simulink model "gm_fourxfour_designfxdpt_givens_vnl"  (R2018b)
settings: Solver=FixedStepDiscrete  StartTime=0.0  StopTime=0.18e-6  RelTol=1e-3
InitFcn:
  | if isempty(which('mylib'))
  |      tmp = fileparts(which(bdroot));
  |      run(fullfile(fileparts(tmp), '5-Utilities', 'addPathsPfcHw.m'));
  | end
  | 
  | data_types_givens
StopFcn:
  | GivensSim_Stop
undefined symbols (not defined in the file or in its folder): f
libraries: simulink x28, mylib x14
(part 1 of 4)
settings Model: Creator=skanaga4  LastModifiedBy=yangli18
settings OptimizationCC: BlockReduction=off  ConditionallyExecuteInputs=off  DefaultParameterBehavior=Inlined
settings DebuggingCC: AlgebraicLoopMsg=error  ArtificialAlgebraicLoopMsg=none  InheritedTsInSrcMsg=none  SingleTaskRateTransMsg=error
settings HardwareCC: ProdBitPerPointer=32  ProdBitPerSizeT=32  ProdBitPerPtrDiffT=32  ProdLargestAtomicFloat=None  ProdIntDivRoundTo=Undefined  ProdEndianess=Unspecified  ProdWordSize=32  ProdHWDeviceType=ASIC/FPGA->ASIC/FPGA  TargetBitPerLong=64  TargetBitPerPointer=64  TargetBitPerSizeT=64  TargetBitPerPtrDiffT=64  TargetLongLongMode=on  TargetIntDivRoundTo=Zero  TargetEndianess=LittleEndian  TargetWordSize=64  TargetHWDeviceType=Custom Processor->MATLAB Host Computer  ProdEqTarget=off

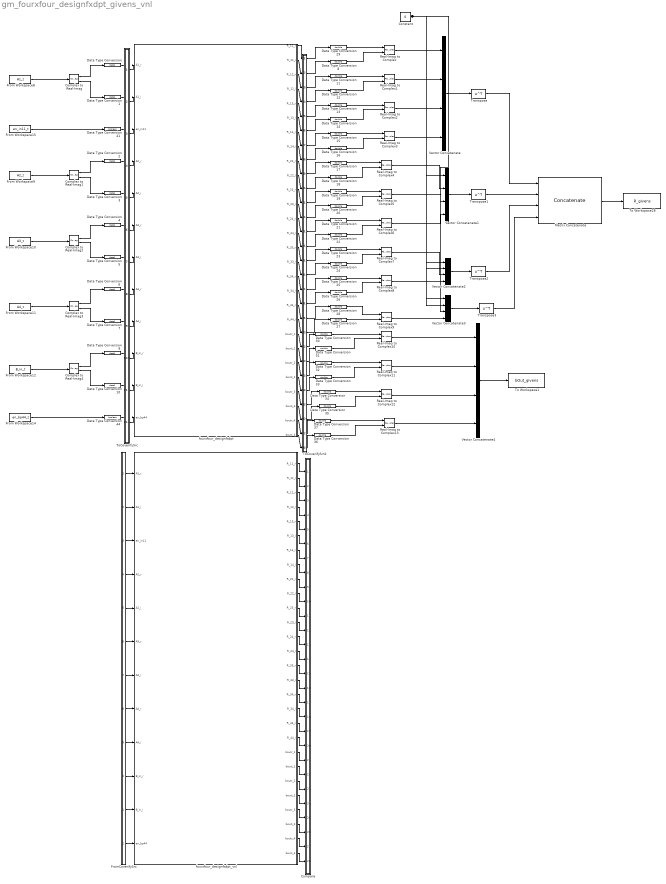
== system gm_fourxfour_designfxdpt_givens_vnl ==
  Compare : Subsystem
      mask Display: disp('')
  Complex to Real-Imag{,1..4} (5 alike) : ComplexToRealImag
  Constant : Constant  Value=0  SampleTime=-1
  Data Type Conversion{,1..7,9..10} (10 alike) : DataTypeConversion  OutDataTypeStr=data1
  Data Type Conversion{8,11..37} (28 alike) : DataTypeConversion  OutDataTypeStr=double
  Data Type Conversion41 : DataTypeConversion  OutDataTypeStr=boolean
  Data Type Conversion44 : DataTypeConversion  OutDataTypeStr=boolean
  From Workspace10 : FromWorkspace  VariableName=A3_t  SampleTime=1/f  Interpolate=off  OutputAfterFinalValue=Holding final value
  From Workspace11 : FromWorkspace  VariableName=A4_t  SampleTime=1/f  Interpolate=off  OutputAfterFinalValue=Holding final value
  From Workspace12 : FromWorkspace  VariableName=B_in_t  SampleTime=1/f  Interpolate=off  OutputAfterFinalValue=Holding final value
  From Workspace14 : FromWorkspace  VariableName=en_bp44_t  SampleTime=1/f  Interpolate=off  OutputAfterFinalValue=Holding final value
  From Workspace15 : FromWorkspace  VariableName=en_in11_t  SampleTime=1/f  Interpolate=off  OutputAfterFinalValue=Holding final value
  From Workspace8 : FromWorkspace  VariableName=A1_t  SampleTime=1/f  Interpolate=off  OutputAfterFinalValue=Holding final value
  From Workspace9 : FromWorkspace  VariableName=A2_t  SampleTime=1/f  Interpolate=off  OutputAfterFinalValue=Holding final value
  FromCoverifySrc : Subsystem
      mask Display: disp('')
  Matrix Concatenate : Concatenate  NumInputs=4  Mode=Multidimensional array
  Real-Imag to Complex{,1..13} (14 alike) : RealImagToComplex
  To Workspace1 : ToWorkspace  VariableName=bOut_givens  SaveFormat=Timeseries  SampleTime=-1
  To Workspace28 : ToWorkspace  VariableName=R_givens  SaveFormat=Timeseries  SampleTime=-1
  ToCoverifySink : Subsystem
      mask Display: disp('')
  ToCoverifySrc : Subsystem
      mask Display: disp('')
  Transpose{,1..3} (4 alike) : Math  Operator=transpose  RndMeth=Zero  SaturateOnIntegerOverflow=on
  Vector Concatenate{,1..4} (5 alike) : Concatenate  NumInputs=4
  fourxfour_designfxdpt : Subsystem
  fourxfour_designfxdpt_vnl : Subsystem
  wires:
  From Workspace8/1 -> Complex to Real-Imag/1
  Complex to Real-Imag/1 -> Data Type Conversion/1
  Complex to Real-Imag/2 -> Data Type Conversion1/1
  From Workspace9/1 -> Complex to Real-Imag1/1
  From Workspace11/1 -> Complex to Real-Imag3/1
  From Workspace10/1 -> Complex to Real-Imag2/1
  Complex to Real-Imag1/1 -> Data Type Conversion2/1
  Complex to Real-Imag1/2 -> Data Type Conversion3/1
  Complex to Real-Imag2/1 -> Data Type Conversion4/1
  Complex to Real-Imag2/2 -> Data Type Conversion5/1
  Complex to Real-Imag3/1 -> Data Type Conversion6/1
  Complex to Real-Imag3/2 -> Data Type Conversion7/1
  From Workspace12/1 -> Complex to Real-Imag4/1
  Complex to Real-Imag4/1 -> Data Type Conversion9/1
  Complex to Real-Imag4/2 -> Data Type Conversion10/1
  From Workspace14/1 -> Data Type Conversion44/1
  From Workspace15/1 -> Data Type Conversion41/1
  Real-Imag to Complex/1 -> Vector Concatenate/1
  Constant/1 -> Vector Concatenate3/3, Vector Concatenate3/2, Vector Concatenate3/1, Vector Concatenate2/2, Vector Concatenate2/1, Vector Concatenate1/1
  Real-Imag to Complex4/1 -> Vector Concatenate1/2
  Real-Imag to Complex9/1 -> Vector Concatenate3/4
  Real-Imag to Complex8/1 -> Vector Concatenate2/4
  Real-Imag to Complex2/1 -> Vector Concatenate/3
  Vector Concatenate/1 -> Transpose/1
  Real-Imag to Complex5/1 -> Vector Concatenate1/3
  Data Type Conversion21/1 -> Real-Imag to Complex6/1
  Data Type Conversion13/1 -> Real-Imag to Complex2/1
  Data Type Conversion12/1 -> Real-Imag to Complex1/2
  Data Type Conversion16/1 -> Real-Imag to Complex3/2
  Data Type Conversion17/1 -> Real-Imag to Complex4/1
  Data Type Conversion18/1 -> Real-Imag to Complex4/2
  Data Type Conversion15/1 -> Real-Imag to Complex3/1
  Data Type Conversion28/1 -> Real-Imag to Complex9/1
  Data Type Conversion29/1 -> Real-Imag to Complex/1
  Matrix Concatenate/1 -> To Workspace28/1
  Vector Concatenate3/1 -> Transpose3/1
  Data Type Conversion23/1 -> Real-Imag to Complex7/1
  Data Type Conversion8/1 -> Real-Imag to Complex/2
  Data Type Conversion24/1 -> Real-Imag to Complex7/2
  Data Type Conversion25/1 -> Real-Imag to Complex8/1
  Transpose/1 -> Matrix Concatenate/1
  Real-Imag to Complex7/1 -> Vector Concatenate2/3
  Transpose3/1 -> Matrix Concatenate/4
  Data Type Conversion19/1 -> Real-Imag to Complex5/1
  Transpose2/1 -> Matrix Concatenate/3
  Data Type Conversion20/1 -> Real-Imag to Complex5/2
  Vector Concatenate1/1 -> Transpose1/1
  Real-Imag to Complex6/1 -> Vector Concatenate1/4
  Transpose1/1 -> Matrix Concatenate/2
  Data Type Conversion22/1 -> Real-Imag to Complex6/2
  Vector Concatenate2/1 -> Transpose2/1
  Data Type Conversion26/1 -> Real-Imag to Complex8/2
  Data Type Conversion11/1 -> Real-Imag to Complex1/1
  Real-Imag to Complex1/1 -> Vector Concatenate/2
  Data Type Conversion14/1 -> Real-Imag to Complex2/2
  Real-Imag to Complex3/1 -> Vector Concatenate/4
  Data Type Conversion27/1 -> Real-Imag to Complex9/2
  Data Type Conversion36/1 -> Real-Imag to Complex13/2
  Data Type Conversion35/1 -> Real-Imag to Complex12/2
  Data Type Conversion31/1 -> Real-Imag to Complex10/2
  Real-Imag to Complex10/1 -> Vector Concatenate4/1
  Real-Imag to Complex11/1 -> Vector Concatenate4/2
  Data Type Conversion34/1 -> Real-Imag to Complex12/1
  Data Type Conversion33/1 -> Real-Imag to Complex11/2
  Data Type Conversion32/1 -> Real-Imag to Complex11/1
  Data Type Conversion37/1 -> Real-Imag to Complex13/1
  Data Type Conversion30/1 -> Real-Imag to Complex10/1
  Real-Imag to Complex12/1 -> Vector Concatenate4/3
  Real-Imag to Complex13/1 -> Vector Concatenate4/4
  Vector Concatenate4/1 -> To Workspace1/1
  ToCoverifySrc/1(out1) -> fourxfour_designfxdpt/1("A1_r ")
  ToCoverifySrc/2(out2) -> fourxfour_designfxdpt/2(A1_i)
  ToCoverifySrc/3(out3) -> fourxfour_designfxdpt/3("en_in11 ")
  ToCoverifySrc/4(out4) -> fourxfour_designfxdpt/4(A2_r)
  ToCoverifySrc/5(out5) -> fourxfour_designfxdpt/5(A2_i)
  ToCoverifySrc/6(out6) -> fourxfour_designfxdpt/6(A3_r)
  ToCoverifySrc/7(out7) -> fourxfour_designfxdpt/7(A3_i)
  ToCoverifySrc/8(out8) -> fourxfour_designfxdpt/8(A4_r)
  ToCoverifySrc/9(out9) -> fourxfour_designfxdpt/9(A4_i)
  ToCoverifySrc/10(out10) -> fourxfour_designfxdpt/10(B_in_r)
  ToCoverifySrc/11(out11) -> fourxfour_designfxdpt/11(B_in_i)
  ToCoverifySrc/12(out12) -> fourxfour_designfxdpt/12(en_bp44)
  fourxfour_designfxdpt/1(R_11_r) -> ToCoverifySink/1(in1)
  fourxfour_designfxdpt/2(R_11_i) -> ToCoverifySink/2(in2)
  fourxfour_designfxdpt/3(R_12_r) -> ToCoverifySink/3(in3)
  fourxfour_designfxdpt/4(R_12_i) -> ToCoverifySink/4(in4)
  fourxfour_designfxdpt/5(R_13_r) -> ToCoverifySink/5(in5)
  fourxfour_designfxdpt/6(R_13_i) -> ToCoverifySink/6(in6)
  fourxfour_designfxdpt/7(R_14_r) -> ToCoverifySink/7(in7)
  fourxfour_designfxdpt/8(R_14_i) -> ToCoverifySink/8(in8)
  fourxfour_designfxdpt/9(R_22_r) -> ToCoverifySink/9(in9)
  fourxfour_designfxdpt/10(R_22_i) -> ToCoverifySink/10(in10)
  fourxfour_designfxdpt/11(R_23_r) -> ToCoverifySink/11(in11)
  fourxfour_designfxdpt/12(R_23_i) -> ToCoverifySink/12(in12)
  fourxfour_designfxdpt/13(R_24_r) -> ToCoverifySink/13(in13)
  fourxfour_designfxdpt/14(R_24_i) -> ToCoverifySink/14(in14)
  fourxfour_designfxdpt/15(R_33_r) -> ToCoverifySink/15(in15)
  fourxfour_designfxdpt/16(R_33_i) -> ToCoverifySink/16(in16)
  fourxfour_designfxdpt/17(R_34_r) -> ToCoverifySink/17(in17)
  fourxfour_designfxdpt/18(R_34_i) -> ToCoverifySink/18(in18)
  fourxfour_designfxdpt/19(R_44_r) -> ToCoverifySink/19(in19)
  fourxfour_designfxdpt/20(R_44_i) -> ToCoverifySink/20(in20)
  fourxfour_designfxdpt/21(boutr_1) -> ToCoverifySink/21(in21)
  fourxfour_designfxdpt/22(bouti_1) -> ToCoverifySink/22(in22)
  fourxfour_designfxdpt/23(boutr_2) -> ToCoverifySink/23(in23)
  fourxfour_designfxdpt/24(bouti_2) -> ToCoverifySink/24(in24)
  fourxfour_designfxdpt/25(boutr_3) -> ToCoverifySink/25(in25)
  fourxfour_designfxdpt/26(bouti_3) -> ToCoverifySink/26(in26)
  fourxfour_designfxdpt/27(boutr_4) -> ToCoverifySink/27(in27)
  fourxfour_designfxdpt/28(bouti_4) -> ToCoverifySink/28(in28)
  Data Type Conversion/1 -> ToCoverifySrc/1(in1)
  Data Type Conversion1/1 -> ToCoverifySrc/2(in2)
  Data Type Conversion41/1 -> ToCoverifySrc/3(in3)
  Data Type Conversion2/1 -> ToCoverifySrc/4(in4)
  Data Type Conversion3/1 -> ToCoverifySrc/5(in5)
  Data Type Conversion4/1 -> ToCoverifySrc/6(in6)
  Data Type Conversion5/1 -> ToCoverifySrc/7(in7)
  Data Type Conversion6/1 -> ToCoverifySrc/8(in8)
  Data Type Conversion7/1 -> ToCoverifySrc/9(in9)
  Data Type Conversion9/1 -> ToCoverifySrc/10(in10)
  Data Type Conversion10/1 -> ToCoverifySrc/11(in11)
  Data Type Conversion44/1 -> ToCoverifySrc/12(in12)
  ToCoverifySink/1(out1) -> Data Type Conversion29/1
  ToCoverifySink/2(out2) -> Data Type Conversion8/1
  ToCoverifySink/3(out3) -> Data Type Conversion11/1
  ToCoverifySink/4(out4) -> Data Type Conversion12/1
  ToCoverifySink/5(out5) -> Data Type Conversion13/1
  ToCoverifySink/6(out6) -> Data Type Conversion14/1
  ToCoverifySink/7(out7) -> Data Type Conversion15/1
  ToCoverifySink/8(out8) -> Data Type Conversion16/1
  ToCoverifySink/9(out9) -> Data Type Conversion17/1
  ToCoverifySink/10(out10) -> Data Type Conversion18/1
  ToCoverifySink/11(out11) -> Data Type Conversion19/1
  ToCoverifySink/12(out12) -> Data Type Conversion20/1
  ToCoverifySink/13(out13) -> Data Type Conversion21/1
  ToCoverifySink/14(out14) -> Data Type Conversion22/1
  ToCoverifySink/15(out15) -> Data Type Conversion23/1
  ToCoverifySink/16(out16) -> Data Type Conversion24/1
  ToCoverifySink/17(out17) -> Data Type Conversion25/1
  ToCoverifySink/18(out18) -> Data Type Conversion26/1
  ToCoverifySink/19(out19) -> Data Type Conversion28/1
  ToCoverifySink/20(out20) -> Data Type Conversion27/1
  ToCoverifySink/21(out21) -> Data Type Conversion30/1
  ToCoverifySink/22(out22) -> Data Type Conversion31/1
  ToCoverifySink/23(out23) -> Data Type Conversion32/1
  ToCoverifySink/24(out24) -> Data Type Conversion33/1
  ToCoverifySink/25(out25) -> Data Type Conversion34/1
  ToCoverifySink/26(out26) -> Data Type Conversion35/1
  ToCoverifySink/27(out27) -> Data Type Conversion37/1
  ToCoverifySink/28(out28) -> Data Type Conversion36/1
  FromCoverifySrc/1(out1) -> fourxfour_designfxdpt_vnl/1("A1_r ")
  FromCoverifySrc/2(out2) -> fourxfour_designfxdpt_vnl/2(A1_i)
  FromCoverifySrc/3(out3) -> fourxfour_designfxdpt_vnl/3("en_in11 ")
  FromCoverifySrc/4(out4) -> fourxfour_designfxdpt_vnl/4(A2_r)
  FromCoverifySrc/5(out5) -> fourxfour_designfxdpt_vnl/5(A2_i)
  FromCoverifySrc/6(out6) -> fourxfour_designfxdpt_vnl/6(A3_r)
  FromCoverifySrc/7(out7) -> fourxfour_designfxdpt_vnl/7(A3_i)
  FromCoverifySrc/8(out8) -> fourxfour_designfxdpt_vnl/8(A4_r)
  FromCoverifySrc/9(out9) -> fourxfour_designfxdpt_vnl/9(A4_i)
  FromCoverifySrc/10(out10) -> fourxfour_designfxdpt_vnl/10(B_in_r)
  FromCoverifySrc/11(out11) -> fourxfour_designfxdpt_vnl/11(B_in_i)
  FromCoverifySrc/12(out12) -> fourxfour_designfxdpt_vnl/12(en_bp44)
  fourxfour_designfxdpt_vnl/1(R_11_r) -> Compare/1(in1)
  fourxfour_designfxdpt_vnl/2(R_11_i) -> Compare/2(in2)
  fourxfour_designfxdpt_vnl/3(R_12_r) -> Compare/3(in3)
  fourxfour_designfxdpt_vnl/4(R_12_i) -> Compare/4(in4)
  fourxfour_designfxdpt_vnl/5(R_13_r) -> Compare/5(in5)
  fourxfour_designfxdpt_vnl/6(R_13_i) -> Compare/6(in6)
  fourxfour_designfxdpt_vnl/7(R_14_r) -> Compare/7(in7)
  fourxfour_designfxdpt_vnl/8(R_14_i) -> Compare/8(in8)
  fourxfour_designfxdpt_vnl/9(R_22_r) -> Compare/9(in9)
  fourxfour_designfxdpt_vnl/10(R_22_i) -> Compare/10(in10)
  fourxfour_designfxdpt_vnl/11(R_23_r) -> Compare/11(in11)
  fourxfour_designfxdpt_vnl/12(R_23_i) -> Compare/12(in12)
  fourxfour_designfxdpt_vnl/13(R_24_r) -> Compare/13(in13)
  fourxfour_designfxdpt_vnl/14(R_24_i) -> Compare/14(in14)
  fourxfour_designfxdpt_vnl/15(R_33_r) -> Compare/15(in15)
  fourxfour_designfxdpt_vnl/16(R_33_i) -> Compare/16(in16)
  fourxfour_designfxdpt_vnl/17(R_34_r) -> Compare/17(in17)
  fourxfour_designfxdpt_vnl/18(R_34_i) -> Compare/18(in18)
  fourxfour_designfxdpt_vnl/19(R_44_r) -> Compare/19(in19)
  fourxfour_designfxdpt_vnl/20(R_44_i) -> Compare/20(in20)
  fourxfour_designfxdpt_vnl/21(boutr_1) -> Compare/21(in21)
  fourxfour_designfxdpt_vnl/22(bouti_1) -> Compare/22(in22)
  fourxfour_designfxdpt_vnl/23(boutr_2) -> Compare/23(in23)
  fourxfour_designfxdpt_vnl/24(bouti_2) -> Compare/24(in24)
  fourxfour_designfxdpt_vnl/25(boutr_3) -> Compare/25(in25)
  fourxfour_designfxdpt_vnl/26(bouti_3) -> Compare/26(in26)
  fourxfour_designfxdpt_vnl/27(boutr_4) -> Compare/27(in27)
  fourxfour_designfxdpt_vnl/28(bouti_4) -> Compare/28(in28)

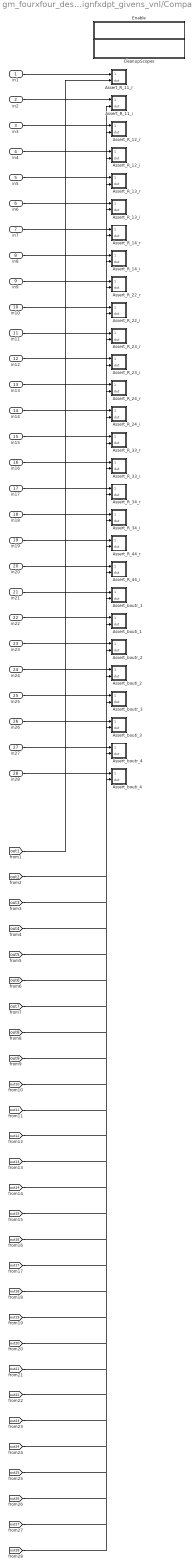
== system gm_fourxfour_designfxdpt_givens_vnl/Compare ==
  in1 : Inport
  in2 : Inport  Port=2
  in3 : Inport  Port=3
  in4 : Inport  Port=4
  in5 : Inport  Port=5
  in6 : Inport  Port=6
  in7 : Inport  Port=7
  in8 : Inport  Port=8
  in9 : Inport  Port=9
  in10 : Inport  Port=10
  in11 : Inport  Port=11
  in12 : Inport  Port=12
  in13 : Inport  Port=13
  in14 : Inport  Port=14
  in15 : Inport  Port=15
  in16 : Inport  Port=16
  in17 : Inport  Port=17
  in18 : Inport  Port=18
  in19 : Inport  Port=19
  in20 : Inport  Port=20
  in21 : Inport  Port=21
  in22 : Inport  Port=22
  in23 : Inport  Port=23
  in24 : Inport  Port=24
  in25 : Inport  Port=25
  in26 : Inport  Port=26
  in27 : Inport  Port=27
  in28 : Inport  Port=28
  Assert_R_11_i : Subsystem
  Assert_R_11_r : Subsystem
  Assert_R_12_i : Subsystem
  Assert_R_12_r : Subsystem
  Assert_R_13_i : Subsystem
  Assert_R_13_r : Subsystem
  Assert_R_14_i : Subsystem
  Assert_R_14_r : Subsystem
  Assert_R_22_i : Subsystem
  Assert_R_22_r : Subsystem
  Assert_R_23_i : Subsystem
  Assert_R_23_r : Subsystem
  Assert_R_24_i : Subsystem
  Assert_R_24_r : Subsystem
  Assert_R_33_i : Subsystem
  Assert_R_33_r : Subsystem
  Assert_R_34_i : Subsystem
  Assert_R_34_r : Subsystem
  Assert_R_44_i : Subsystem
  Assert_R_44_r : Subsystem
  Assert_bouti_1 : Subsystem
  Assert_bouti_2 : Subsystem
  Assert_bouti_3 : Subsystem
  Assert_bouti_4 : Subsystem
  Assert_boutr_1 : Subsystem
  Assert_boutr_2 : Subsystem
  Assert_boutr_3 : Subsystem
  Assert_boutr_4 : Subsystem
  CleanupScopes : Subsystem
      settings: OpenFcn=|
      | blkName = gcb; %self block
      | idx = regexp(blkName, '/CleanupScopes$', 'once');
      | blkParent = blkName(1:idx-1);
      | blks=find_system(blkParent, 'LookUnderMasks', 'all','blocktype', 'Scope');
      | for itr = 1:length(blks)
      | 	 hScopeCfg = get_param(blks{itr},'ScopeConfiguration');
      | 	 hScopeCfg.Visible = ~ hScopeCfg.Visible;
      | end
      | drawnow;
      mask Display: fprintf(message('hdlcoder:cosim:vnl_dblclick').getString());
  Enable : Subsystem
      settings: OpenFcn=|
      | blkName = gcb;
      | idx = regexp(blkName, '/Enable$', 'once');
      | blkParent = blkName(1:idx-1);
      | blks=find_system(blkParent, 'LookUnderMasks', 'all','blocktype', 'Assertion');
      | e = get_param(blks{1}, 'Enabled');
      | if strcmp(e, 'on'), f= 'off';, else, f = 'on';, end
      | for ii=1:length(blks), set_param(blks{ii}, 'Enabled', f);, end
      | set_param(gcb, 'MaskDisplay',['fprintf(message(''hdlcoder:cosim:vnl_dblclick_assertions'',','''',upper(e),'''',').getString())']);
      mask Display: fprintf(message('hdlcoder:cosim:vnl_dblclick_assertions','OFF').getString());
  wires:
  in1/1 -> Assert_R_11_r/1(cosim)
  [out1] -> Assert_R_11_r/2(dut)
  in2/1 -> Assert_R_11_i/1(cosim)
  [out2] -> Assert_R_11_i/2(dut)
  in3/1 -> Assert_R_12_r/1(cosim)
  [out3] -> Assert_R_12_r/2(dut)
  in4/1 -> Assert_R_12_i/1(cosim)
  [out4] -> Assert_R_12_i/2(dut)
  in5/1 -> Assert_R_13_r/1(cosim)
  [out5] -> Assert_R_13_r/2(dut)
  in6/1 -> Assert_R_13_i/1(cosim)
  [out6] -> Assert_R_13_i/2(dut)
  in7/1 -> Assert_R_14_r/1(cosim)
  [out7] -> Assert_R_14_r/2(dut)
  in8/1 -> Assert_R_14_i/1(cosim)
  [out8] -> Assert_R_14_i/2(dut)
  in9/1 -> Assert_R_22_r/1(cosim)
  [out9] -> Assert_R_22_r/2(dut)
  in10/1 -> Assert_R_22_i/1(cosim)
  [out10] -> Assert_R_22_i/2(dut)
  in11/1 -> Assert_R_23_r/1(cosim)
  [out11] -> Assert_R_23_r/2(dut)
  in12/1 -> Assert_R_23_i/1(cosim)
  [out12] -> Assert_R_23_i/2(dut)
  in13/1 -> Assert_R_24_r/1(cosim)
  [out13] -> Assert_R_24_r/2(dut)
  in14/1 -> Assert_R_24_i/1(cosim)
  [out14] -> Assert_R_24_i/2(dut)
  in15/1 -> Assert_R_33_r/1(cosim)
  [out15] -> Assert_R_33_r/2(dut)
  in16/1 -> Assert_R_33_i/1(cosim)
  [out16] -> Assert_R_33_i/2(dut)
  in17/1 -> Assert_R_34_r/1(cosim)
  [out17] -> Assert_R_34_r/2(dut)
  in18/1 -> Assert_R_34_i/1(cosim)
  [out18] -> Assert_R_34_i/2(dut)
  in19/1 -> Assert_R_44_r/1(cosim)
  [out19] -> Assert_R_44_r/2(dut)
  in20/1 -> Assert_R_44_i/1(cosim)
  [out20] -> Assert_R_44_i/2(dut)
  in21/1 -> Assert_boutr_1/1(cosim)
  [out21] -> Assert_boutr_1/2(dut)
  in22/1 -> Assert_bouti_1/1(cosim)
  [out22] -> Assert_bouti_1/2(dut)
  in23/1 -> Assert_boutr_2/1(cosim)
  [out23] -> Assert_boutr_2/2(dut)
  in24/1 -> Assert_bouti_2/1(cosim)
  [out24] -> Assert_bouti_2/2(dut)
  in25/1 -> Assert_boutr_3/1(cosim)
  [out25] -> Assert_boutr_3/2(dut)
  in26/1 -> Assert_bouti_3/1(cosim)
  [out26] -> Assert_bouti_3/2(dut)
  in27/1 -> Assert_boutr_4/1(cosim)
  [out27] -> Assert_boutr_4/2(dut)
  in28/1 -> Assert_bouti_4/1(cosim)
  [out28] -> Assert_bouti_4/2(dut)

== system gm_fourxfour_designfxdpt_givens_vnl/FromCoverifySrc ==
  out1 : Outport
  out2 : Outport  Port=2
  out3 : Outport  Port=3
  out4 : Outport  Port=4
  out5 : Outport  Port=5
  out6 : Outport  Port=6
  out7 : Outport  Port=7
  out8 : Outport  Port=8
  out9 : Outport  Port=9
  out10 : Outport  Port=10
  out11 : Outport  Port=11
  out12 : Outport  Port=12
  wires:
  [in1] -> out1/1
  [in2] -> out2/1
  [in3] -> out3/1
  [in4] -> out4/1
  [in5] -> out5/1
  [in6] -> out6/1
  [in7] -> out7/1
  [in8] -> out8/1
  [in9] -> out9/1
  [in10] -> out10/1
  [in11] -> out11/1
  [in12] -> out12/1

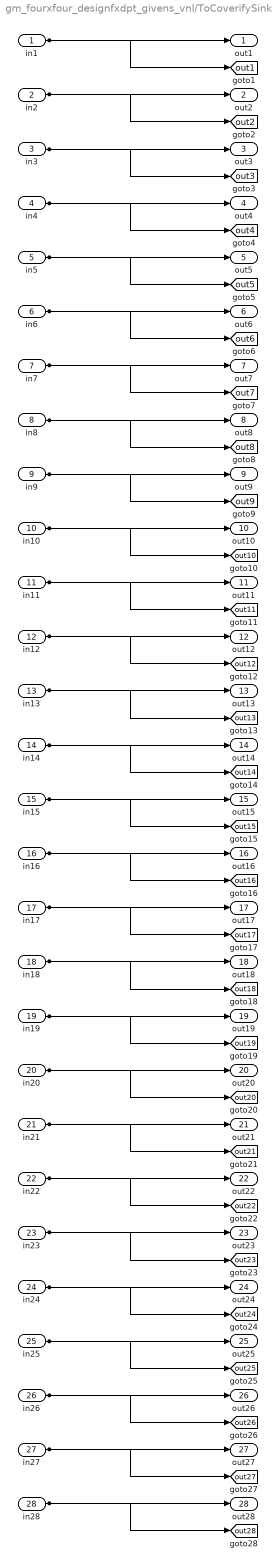
== system gm_fourxfour_designfxdpt_givens_vnl/ToCoverifySink ==
  in1 : Inport
  in2 : Inport  Port=2
  in3 : Inport  Port=3
  in4 : Inport  Port=4
  in5 : Inport  Port=5
  in6 : Inport  Port=6
  in7 : Inport  Port=7
  in8 : Inport  Port=8
  in9 : Inport  Port=9
  in10 : Inport  Port=10
  in11 : Inport  Port=11
  in12 : Inport  Port=12
  in13 : Inport  Port=13
  in14 : Inport  Port=14
  in15 : Inport  Port=15
  in16 : Inport  Port=16
  in17 : Inport  Port=17
  in18 : Inport  Port=18
  in19 : Inport  Port=19
  in20 : Inport  Port=20
  in21 : Inport  Port=21
  in22 : Inport  Port=22
  in23 : Inport  Port=23
  in24 : Inport  Port=24
  in25 : Inport  Port=25
  in26 : Inport  Port=26
  in27 : Inport  Port=27
  in28 : Inport  Port=28
  out1 : Outport
  out2 : Outport  Port=2
  out3 : Outport  Port=3
  out4 : Outport  Port=4
  out5 : Outport  Port=5
  out6 : Outport  Port=6
  out7 : Outport  Port=7
  out8 : Outport  Port=8
  out9 : Outport  Port=9
  out10 : Outport  Port=10
  out11 : Outport  Port=11
  out12 : Outport  Port=12
  out13 : Outport  Port=13
  out14 : Outport  Port=14
  out15 : Outport  Port=15
  out16 : Outport  Port=16
  out17 : Outport  Port=17
  out18 : Outport  Port=18
  out19 : Outport  Port=19
  out20 : Outport  Port=20
  out21 : Outport  Port=21
  out22 : Outport  Port=22
  out23 : Outport  Port=23
  out24 : Outport  Port=24
  out25 : Outport  Port=25
  out26 : Outport  Port=26
  out27 : Outport  Port=27
  out28 : Outport  Port=28
  tag scope: out10=global, out11=global, out12=global, out13=global, out14=global, out15=global, out16=global, out17=global, out18=global, out19=global, out1=global, out20=global, out21=global, out22=global, out23=global, out24=global, out25=global, out26=global, out27=global, out28=global, out2=global, out3=global, out4=global, out5=global, out6=global, out7=global, out8=global, out9=global
  wires:
  in1/1 -> out1/1, [out1]
  in2/1 -> out2/1, [out2]
  in3/1 -> out3/1, [out3]
  in4/1 -> out4/1, [out4]
  in5/1 -> out5/1, [out5]
  in6/1 -> out6/1, [out6]
  in7/1 -> out7/1, [out7]
  in8/1 -> out8/1, [out8]
  in9/1 -> out9/1, [out9]
  in10/1 -> out10/1, [out10]
  in11/1 -> out11/1, [out11]
  in12/1 -> out12/1, [out12]
  in13/1 -> out13/1, [out13]
  in14/1 -> out14/1, [out14]
  in15/1 -> out15/1, [out15]
  in16/1 -> out16/1, [out16]
  in17/1 -> out17/1, [out17]
  in18/1 -> out18/1, [out18]
  in19/1 -> out19/1, [out19]
  in20/1 -> out20/1, [out20]
  in21/1 -> out21/1, [out21]
  in22/1 -> out22/1, [out22]
  in23/1 -> out23/1, [out23]
  in24/1 -> out24/1, [out24]
  in25/1 -> out25/1, [out25]
  in26/1 -> out26/1, [out26]
  in27/1 -> out27/1, [out27]
  in28/1 -> out28/1, [out28]

== system gm_fourxfour_designfxdpt_givens_vnl/ToCoverifySrc ==
  in1 : Inport
  in2 : Inport  Port=2
  in3 : Inport  Port=3
  in4 : Inport  Port=4
  in5 : Inport  Port=5
  in6 : Inport  Port=6
  in7 : Inport  Port=7
  in8 : Inport  Port=8
  in9 : Inport  Port=9
  in10 : Inport  Port=10
  in11 : Inport  Port=11
  in12 : Inport  Port=12
  out1 : Outport
  out2 : Outport  Port=2
  out3 : Outport  Port=3
  out4 : Outport  Port=4
  out5 : Outport  Port=5
  out6 : Outport  Port=6
  out7 : Outport  Port=7
  out8 : Outport  Port=8
  out9 : Outport  Port=9
  out10 : Outport  Port=10
  out11 : Outport  Port=11
  out12 : Outport  Port=12
  tag scope: in10=global, in11=global, in12=global, in1=global, in2=global, in3=global, in4=global, in5=global, in6=global, in7=global, in8=global, in9=global
  wires:
  in1/1 -> out1/1, [in1]
  in2/1 -> out2/1, [in2]
  in3/1 -> out3/1, [in3]
  in4/1 -> out4/1, [in4]
  in5/1 -> out5/1, [in5]
  in6/1 -> out6/1, [in6]
  in7/1 -> out7/1, [in7]
  in8/1 -> out8/1, [in8]
  in9/1 -> out9/1, [in9]
  in10/1 -> out10/1, [in10]
  in11/1 -> out11/1, [in11]
  in12/1 -> out12/1, [in12]

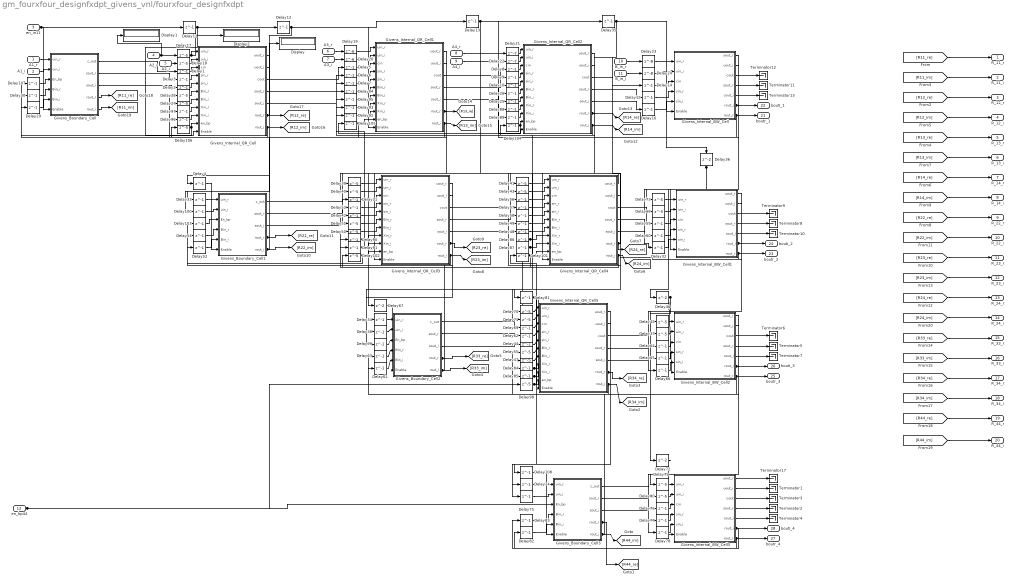
== system gm_fourxfour_designfxdpt_givens_vnl/fourxfour_designfxdpt ==
  "A1_r " : Inport  OutDataTypeStr=fixdt(1, 24, 14)  PortDimensions=1  SampleTime=1e-08
  A1_i : Inport  Port=2  OutDataTypeStr=fixdt(1, 24, 14)  PortDimensions=1  SampleTime=1e-08
  "en_in11 " : Inport  Port=3  OutDataTypeStr=boolean  PortDimensions=1  SampleTime=1e-08
  A2_r : Inport  Port=4  OutDataTypeStr=fixdt(1, 24, 14)  PortDimensions=1  SampleTime=1e-08
  A2_i : Inport  Port=5  OutDataTypeStr=fixdt(1, 24, 14)  PortDimensions=1  SampleTime=1e-08
  A3_r : Inport  Port=6  OutDataTypeStr=fixdt(1, 24, 14)  PortDimensions=1  SampleTime=1e-08
  A3_i : Inport  Port=7  OutDataTypeStr=fixdt(1, 24, 14)  PortDimensions=1  SampleTime=1e-08
  A4_r : Inport  Port=8  OutDataTypeStr=fixdt(1, 24, 14)  PortDimensions=1  SampleTime=1e-08
  A4_i : Inport  Port=9  OutDataTypeStr=fixdt(1, 24, 14)  PortDimensions=1  SampleTime=1e-08
  B_in_r : Inport  Port=10  OutDataTypeStr=fixdt(1, 24, 14)  PortDimensions=1  SampleTime=1e-08
  B_in_i : Inport  Port=11  OutDataTypeStr=fixdt(1, 24, 14)  PortDimensions=1  SampleTime=1e-08
  en_bp44 : Inport  Port=12  OutDataTypeStr=boolean  PortDimensions=1  SampleTime=1e-08
  Delay{1..16,25..26,29..35,38,42,44,48..49,52..54,56..66,69,74..78,81..97,99..101,103..105,107..108} (75 alike) : Delay  DelayLength=1  InitialCondition=0
  Delay{17..18,27..28,37,39..41,43,45,47,50..51,55,68,70..71,73,79..80,98,102,106} (23 alike) : Delay  DelayLength=5  InitialCondition=0
  Delay19 : Delay  DelayLength=6  InitialCondition=0
  Delay20 : Delay  DelayLength=6  InitialCondition=0
  Delay21 : Delay  DelayLength=7  InitialCondition=0
  Delay22 : Delay  DelayLength=7  InitialCondition=0
  Delay23 : Delay  DelayLength=8  InitialCondition=0
  Delay24 : Delay  DelayLength=8  InitialCondition=0
  Delay{36,46,67,72} (4 alike) : Delay  InitialCondition=0
  Display : Display
  Display1 : Display
  Display2 : Display
  Givens_Boundary_Cell : Subsystem
  Givens_Boundary_Cell1 : Subsystem
  Givens_Boundary_Cell2 : Subsystem
  Givens_Boundary_Cell3 : Subsystem
  Givens_Internal_BW_Cell : Subsystem
  Givens_Internal_BW_Cell1 : Subsystem
  Givens_Internal_BW_Cell2 : Subsystem
  Givens_Internal_BW_Cell3 : Subsystem
  Givens_Internal_QR_Cell : Subsystem
  Givens_Internal_QR_Cell1 : Subsystem
  Givens_Internal_QR_Cell2 : Subsystem
  Givens_Internal_QR_Cell3 : Subsystem
  Givens_Internal_QR_Cell4 : Subsystem
  Givens_Internal_QR_Cell5 : Subsystem
  Terminator{1..13,17} (14 alike) : Terminator
  R_11_r : Outport
  R_11_i : Outport  Port=2
  R_12_r : Outport  Port=3
  R_12_i : Outport  Port=4
  R_13_r : Outport  Port=5
  R_13_i : Outport  Port=6
  R_14_r : Outport  Port=7
  R_14_i : Outport  Port=8
  R_22_r : Outport  Port=9
  R_22_i : Outport  Port=10
  R_23_r : Outport  Port=11
  R_23_i : Outport  Port=12
  R_24_r : Outport  Port=13
  R_24_i : Outport  Port=14
  R_33_r : Outport  Port=15
  R_33_i : Outport  Port=16
  R_34_r : Outport  Port=17
  R_34_i : Outport  Port=18
  R_44_r : Outport  Port=19
  R_44_i : Outport  Port=20
  boutr_1 : Outport  Port=21
  bouti_1 : Outport  Port=22
  boutr_2 : Outport  Port=23
  bouti_2 : Outport  Port=24
  boutr_3 : Outport  Port=25
  bouti_3 : Outport  Port=26
  boutr_4 : Outport  Port=27
  bouti_4 : Outport  Port=28
  wires:
  Givens_Boundary_Cell/3(sout_i) -> Delay2/1
  Givens_Boundary_Cell/2(sout_r) -> Delay3/1
  Givens_Boundary_Cell/1(c_out) -> Delay1/1
  Givens_Internal_QR_Cell/5(sout_i) -> Delay7/1
  Givens_Internal_QR_Cell/4(sout_r) -> Delay6/1
  Givens_Internal_QR_Cell/3(cout) -> Delay5/1
  Givens_Internal_QR_Cell/2(uout_i) -> Delay100/1
  Givens_Internal_QR_Cell/1(uout_r) -> Delay33/1
  Delay1/1 -> Givens_Internal_QR_Cell/3(cin)
  Delay3/1 -> Givens_Internal_QR_Cell/4(sin_r)
  Delay2/1 -> Givens_Internal_QR_Cell/5(sin_i)
  Givens_Internal_QR_Cell1/5(sout_i) -> Delay10/1
  Givens_Internal_QR_Cell1/4(sout_r) -> Delay9/1
  Givens_Internal_QR_Cell1/3(cout) -> Delay8/1
  Givens_Internal_QR_Cell1/2(uout_i) -> Delay40/1
  Givens_Internal_QR_Cell1/1(uout_r) -> Delay39/1
  Delay5/1 -> Givens_Internal_QR_Cell1/3(cin)
  Delay6/1 -> Givens_Internal_QR_Cell1/4(sin_r)
  Delay7/1 -> Givens_Internal_QR_Cell1/5(sin_i)
  Givens_Internal_QR_Cell2/5(sout_i) -> Delay16/1
  Givens_Internal_QR_Cell2/4(sout_r) -> Delay15/1
  Givens_Internal_QR_Cell2/3(cout) -> Delay14/1
  Givens_Internal_QR_Cell2/2(uout_i) -> Delay43/1
  Givens_Internal_QR_Cell2/1(uout_r) -> Delay41/1
  Delay8/1 -> Givens_Internal_QR_Cell2/3(cin)
  Delay9/1 -> Givens_Internal_QR_Cell2/4(sin_r)
  Delay10/1 -> Givens_Internal_QR_Cell2/5(sin_i)
  Givens_Internal_BW_Cell/2(uout_i) -> Delay68/1
  Givens_Internal_BW_Cell/1(uout_r) -> Delay73/1
  Delay14/1 -> Givens_Internal_BW_Cell/3(cin)
  Delay15/1 -> Givens_Internal_BW_Cell/4(sin_r)
  Delay16/1 -> Givens_Internal_BW_Cell/5(sin_i)
  Delay26/1 -> Givens_Internal_QR_Cell2/6(Bin_r)
  Delay25/1 -> Givens_Internal_QR_Cell2/7(Bin_i)
  Givens_Boundary_Cell3/3(sout_i) -> Delay78/1
  Givens_Boundary_Cell3/2(sout_r) -> Delay77/1
  Givens_Boundary_Cell3/1(c_out) -> Delay76/1
  Givens_Internal_QR_Cell5/5(sout_i) -> Delay66/1
  Givens_Internal_QR_Cell5/4(sout_r) -> Delay65/1
  Givens_Internal_QR_Cell5/3(cout) -> Delay64/1
  Givens_Internal_QR_Cell5/2(uout_i) -> Delay75/1
  Givens_Internal_QR_Cell5/1(uout_r) -> Delay74/1
  Givens_Internal_QR_Cell4/5(sout_i) -> Delay32/1
  Givens_Internal_QR_Cell4/4(sout_r) -> Delay60/1
  Givens_Internal_QR_Cell4/3(cout) -> Delay59/1
  Givens_Internal_QR_Cell4/2(uout_i) -> Delay71/1
  Givens_Internal_QR_Cell4/1(uout_r) -> Delay70/1
  Delay41/1 -> Givens_Internal_QR_Cell4/1(uin_r)
  Delay43/1 -> Givens_Internal_QR_Cell4/2(uin_i)
  Givens_Internal_QR_Cell3/5(sout_i) -> Delay58/1
  Givens_Internal_QR_Cell3/4(sout_r) -> Delay57/1
  Givens_Internal_QR_Cell3/3(cout) -> Delay56/1
  Givens_Internal_QR_Cell3/2(uout_i) -> Delay38/1
  Givens_Internal_QR_Cell3/1(uout_r) -> Delay34/1
  Delay39/1 -> Givens_Internal_QR_Cell3/1(uin_r)
  Delay40/1 -> Givens_Internal_QR_Cell3/2(uin_i)
  Givens_Boundary_Cell1/3(sout_i) -> Delay42/1
  Givens_Boundary_Cell1/2(sout_r) -> Delay53/1
  Givens_Boundary_Cell1/1(c_out) -> Delay31/1
  Delay33/1 -> Givens_Boundary_Cell1/1(uin_r)
  Delay100/1 -> Givens_Boundary_Cell1/2(uin_i)
  Delay54/1 -> Givens_Boundary_Cell1/4(Bin_r)
  Delay52/1 -> Givens_Boundary_Cell1/5(Bin_i)
  Delay31/1 -> Givens_Internal_QR_Cell3/3(cin)
  Delay53/1 -> Givens_Internal_QR_Cell3/4(sin_r)
  Delay42/1 -> Givens_Internal_QR_Cell3/5(sin_i)
  Delay51/1 -> Givens_Internal_QR_Cell3/6(Bin_r)
  Delay50/1 -> Givens_Internal_QR_Cell3/7(Bin_i)
  Givens_Boundary_Cell2/3(sout_i) -> Delay44/1
  Givens_Boundary_Cell2/2(sout_r) -> Delay62/1
  Givens_Boundary_Cell2/1(c_out) -> Delay69/1
  Delay34/1 -> Givens_Boundary_Cell2/1(uin_r)
  Delay38/1 -> Givens_Boundary_Cell2/2(uin_i)
  Delay63/1 -> Givens_Boundary_Cell2/4(Bin_r)
  Delay61/1 -> Givens_Boundary_Cell2/5(Bin_i)
  Delay90/1 -> Givens_Internal_QR_Cell3/8(Xin_r), Delay93/1
  Delay91/1 -> Givens_Internal_QR_Cell3/9(Xin_i), Delay92/1
  Delay56/1 -> Givens_Internal_QR_Cell4/3(cin)
  Delay57/1 -> Givens_Internal_QR_Cell4/4(sin_r)
  Delay58/1 -> Givens_Internal_QR_Cell4/5(sin_i)
  Givens_Internal_BW_Cell1/2(uout_i) -> Delay37/1
  Givens_Internal_BW_Cell1/1(uout_r) -> Delay45/1
  Delay73/1 -> Givens_Internal_BW_Cell1/1(uin_r)
  Delay68/1 -> Givens_Internal_BW_Cell1/2(uin_i)
  Delay59/1 -> Givens_Internal_BW_Cell1/3(cin)
  Delay60/1 -> Givens_Internal_BW_Cell1/4(sin_r)
  Delay32/1 -> Givens_Internal_BW_Cell1/5(sin_i)
  Delay49/1 -> Givens_Internal_QR_Cell4/6(Bin_r)
  Delay48/1 -> Givens_Internal_QR_Cell4/7(Bin_i)
  Delay86/1 -> Givens_Internal_QR_Cell4/8(Xin_r), Delay88/1
  Delay84/1 -> Givens_Internal_QR_Cell5/8(Xin_r), Delay86/1
  Delay85/1 -> Givens_Internal_QR_Cell5/9(Xin_i), Delay87/1
  Delay87/1 -> Givens_Internal_QR_Cell4/9(Xin_i), Delay89/1
  Delay70/1 -> Givens_Internal_QR_Cell5/1(uin_r)
  Delay71/1 -> Givens_Internal_QR_Cell5/2(uin_i)
  Delay69/1 -> Givens_Internal_QR_Cell5/3(cin)
  Delay62/1 -> Givens_Internal_QR_Cell5/4(sin_r)
  Delay44/1 -> Givens_Internal_QR_Cell5/5(sin_i)
  Givens_Internal_BW_Cell2/2(uout_i) -> Delay80/1
  Givens_Internal_BW_Cell2/1(uout_r) -> Delay79/1
  Delay45/1 -> Givens_Internal_BW_Cell2/1(uin_r)
  Delay37/1 -> Givens_Internal_BW_Cell2/2(uin_i)
  Delay64/1 -> Givens_Internal_BW_Cell2/3(cin)
  Delay65/1 -> Givens_Internal_BW_Cell2/4(sin_r)
  Delay66/1 -> Givens_Internal_BW_Cell2/5(sin_i)
  Delay55/1 -> Givens_Internal_QR_Cell5/6(Bin_r)
  Delay47/1 -> Givens_Internal_QR_Cell5/7(Bin_i)
  Delay74/1 -> Givens_Boundary_Cell3/1(uin_r)
  Delay75/1 -> Givens_Boundary_Cell3/2(uin_i)
  Delay79/1 -> Givens_Internal_BW_Cell3/1(uin_r)
  Delay80/1 -> Givens_Internal_BW_Cell3/2(uin_i)
  Delay76/1 -> Givens_Internal_BW_Cell3/3(cin)
  Delay77/1 -> Givens_Internal_BW_Cell3/4(sin_r)
  Delay78/1 -> Givens_Internal_BW_Cell3/5(sin_i)
  Delay83/1 -> Givens_Boundary_Cell3/4(Bin_r)
  Delay82/1 -> Givens_Boundary_Cell3/5(Bin_i)
  Delay88/1 -> Givens_Internal_QR_Cell2/8(Xin_r)
  Delay89/1 -> Givens_Internal_QR_Cell2/9(Xin_i)
  Delay94/1 -> Givens_Internal_QR_Cell1/6(Bin_r)
  Delay95/1 -> Givens_Internal_QR_Cell1/7(Bin_i)
  Delay93/1 -> Givens_Internal_QR_Cell1/8(Xin_r)
  Delay92/1 -> Givens_Internal_QR_Cell1/9(Xin_i)
  Delay28/1 -> Givens_Internal_QR_Cell/6(Bin_r)
  Delay27/1 -> Givens_Internal_QR_Cell/7(Bin_i)
  Delay97/1 -> Givens_Internal_QR_Cell/8(Xin_r)
  Delay96/1 -> Givens_Internal_QR_Cell/9(Xin_i)
  Delay30/1 -> Givens_Boundary_Cell/4(Bin_r)
  Delay29/1 -> Givens_Boundary_Cell/5(Bin_i)
  Givens_Internal_QR_Cell5/7(rout_i) -> Delay61/1, [R34_im]
  Givens_Internal_QR_Cell5/6(rout_r) -> Delay63/1, [R34_re]
  Givens_Internal_QR_Cell4/7(rout_i) -> Delay50/1, [R24_im]
  Givens_Internal_QR_Cell4/6(rout_r) -> Delay51/1, [R24_re]
  Givens_Internal_QR_Cell3/7(rout_i) -> Delay52/1, [R23_im]
  Givens_Internal_QR_Cell3/6(rout_r) -> Delay54/1, [R23_re]
  Givens_Internal_QR_Cell2/7(rout_i) -> Delay95/1, [R14_im]
  Givens_Internal_QR_Cell2/6(rout_r) -> Delay94/1, [R14_re]
  Givens_Internal_QR_Cell1/7(rout_i) -> Delay27/1, [R13_im]
  Givens_Internal_QR_Cell1/6(rout_r) -> Delay28/1, [R13_re]
  Givens_Internal_QR_Cell/7(rout_i) -> Delay29/1, [R12_im]
  Givens_Internal_QR_Cell/6(rout_r) -> Delay30/1, Display/1, [R12_re]
  Givens_Internal_BW_Cell3/7(rout_r) -> Delay83/1, boutr_4/1
  Givens_Internal_BW_Cell3/6(rout_i) -> Delay82/1, bouti_4/1
  Givens_Internal_BW_Cell3/5(sout_i) -> Terminator4/1
  Givens_Internal_BW_Cell3/4(sout_r) -> Terminator2/1
  Givens_Internal_BW_Cell3/3(cout) -> Terminator3/1
  Givens_Internal_BW_Cell3/2(uout_i) -> Terminator1/1
  Givens_Internal_BW_Cell3/1(uout_r) -> Terminator17/1
  Givens_Internal_BW_Cell2/7(rout_r) -> Delay55/1, boutr_3/1
  Givens_Internal_BW_Cell2/6(rout_i) -> Delay47/1, bouti_3/1
  Givens_Internal_BW_Cell2/5(sout_i) -> Terminator7/1
  Givens_Internal_BW_Cell2/4(sout_r) -> Terminator5/1
  Givens_Internal_BW_Cell2/3(cout) -> Terminator6/1
  Givens_Internal_BW_Cell1/7(rout_r) -> Delay49/1, boutr_2/1
  Givens_Internal_BW_Cell1/6(rout_i) -> Delay48/1, bouti_2/1
  Givens_Internal_BW_Cell1/5(sout_i) -> Terminator10/1
  Givens_Internal_BW_Cell1/4(sout_r) -> Terminator8/1
  Givens_Internal_BW_Cell1/3(cout) -> Terminator9/1
  Givens_Internal_BW_Cell/7(rout_r) -> Delay26/1, boutr_1/1
  Givens_Internal_BW_Cell/6(rout_i) -> Delay25/1, bouti_1/1
  Givens_Internal_BW_Cell/5(sout_i) -> Terminator13/1
  Givens_Internal_BW_Cell/4(sout_r) -> Terminator11/1
  Givens_Internal_BW_Cell/3(cout) -> Terminator12/1
  Givens_Boundary_Cell3/5(rout_i) -> Delay85/1, [R44_im]
  Givens_Boundary_Cell3/4(rout_r) -> Delay84/1, [R44_re]
  Givens_Boundary_Cell2/5(rout_i) -> Delay91/1, [R33_im]
  Givens_Boundary_Cell2/4(rout_r) -> Delay90/1, [R33_re]
  Givens_Boundary_Cell1/5(rout_i) -> Delay96/1, [R22_im]
  Givens_Boundary_Cell1/4(rout_r) -> Delay97/1, [R22_re]
  Givens_Boundary_Cell/5(rout_i) -> [R11_im]
  Givens_Boundary_Cell/4(rout_r) -> [R11_re]
  [R14_im] -> R_14_i/1
  [R22_re] -> R_22_r/1
  [R13_im] -> R_13_i/1
  [R14_re] -> R_14_r/1
  [R12_im] -> R_12_i/1
  [R13_re] -> R_13_r/1
  [R11_im] -> R_11_i/1
  [R24_im] -> R_24_i/1
  [R12_re] -> R_12_r/1
  [R44_im] -> R_44_i/1
  [R44_re] -> R_44_r/1
  [R34_im] -> R_34_i/1
  [R34_re] -> R_34_r/1
  [R33_im] -> R_33_i/1
  [R33_re] -> R_33_r/1
  [R23_im] -> R_23_i/1
  [R24_re] -> R_24_r/1
  [R22_im] -> R_22_i/1
  [R23_re] -> R_23_r/1
  [R11_re] -> R_11_r/1
  Delay99/1 -> Givens_Boundary_Cell2/3(En_bp)
  Delay98/1 -> Givens_Internal_QR_Cell5/10(en_bp), Delay101/1, Delay99/1
  Delay81/1 -> Givens_Internal_QR_Cell5/11(Enable), Delay108/1
  Delay72/1 -> Givens_Internal_BW_Cell3/6(Enable)
  Delay67/1 -> Givens_Boundary_Cell2/6(Enable)
  Delay46/1 -> Givens_Internal_BW_Cell2/6(Enable), Delay72/1
  Delay4/1 -> Givens_Boundary_Cell1/6(Enable)
  Delay36/1 -> Givens_Internal_BW_Cell1/6(Enable), Delay46/1
  Delay35/1 -> Givens_Internal_BW_Cell/6(Enable), Givens_Internal_QR_Cell4/11(Enable), Delay36/1, Delay67/1, Delay81/1
  Delay24/1 -> Givens_Internal_BW_Cell/2(uin_i)
  Delay23/1 -> Givens_Internal_BW_Cell/1(uin_r)
  Delay22/1 -> Givens_Internal_QR_Cell2/2(uin_i)
  Delay21/1 -> Givens_Internal_QR_Cell2/1(uin_r)
  Delay20/1 -> Givens_Internal_QR_Cell1/2(uin_i)
  Delay19/1 -> Givens_Internal_QR_Cell1/1(uin_r)
  Delay18/1 -> Givens_Internal_QR_Cell/2(uin_i)
  Delay17/1 -> Givens_Internal_QR_Cell/1(uin_r), Display2/1
  Delay13/1 -> Givens_Internal_QR_Cell3/11(Enable), Givens_Internal_QR_Cell2/11(Enable), Delay35/1
  Delay12/1 -> Givens_Internal_QR_Cell1/11(Enable), Delay13/1, Delay4/1
  Delay11/1 -> Givens_Internal_QR_Cell/11(Enable), Delay12/1
  Delay108/1 -> Givens_Boundary_Cell3/6(Enable)
  Delay107/1 -> Givens_Boundary_Cell/3(En_bp)
  Delay106/1 -> Givens_Internal_QR_Cell/10(en_bp), Delay107/1
  Delay105/1 -> Givens_Internal_QR_Cell1/10(en_bp), Delay106/1
  Delay104/1 -> Givens_Internal_QR_Cell2/10(en_bp), Delay105/1
  Delay103/1 -> Givens_Boundary_Cell1/3(En_bp)
  Delay102/1 -> Givens_Internal_QR_Cell3/10(en_bp), Delay103/1
  Delay101/1 -> Givens_Internal_QR_Cell4/10(en_bp), Delay102/1, Delay104/1
  en_bp44/1 -> Givens_Boundary_Cell3/3(En_bp), Delay98/1
  B_in_i/1 -> Delay24/1
  B_in_r/1 -> Delay23/1
  A4_i/1 -> Delay22/1
  A4_r/1 -> Delay21/1
  A3_i/1 -> Delay20/1
  A3_r/1 -> Delay19/1
  A2_i/1 -> Delay18/1
  A2_r/1 -> Delay17/1, Display1/1
  "en_in11 "/1 -> Givens_Boundary_Cell/6(Enable), Delay11/1
  A1_i/1 -> Givens_Boundary_Cell/2(uin_i)
  "A1_r "/1 -> Givens_Boundary_Cell/1(uin_r)

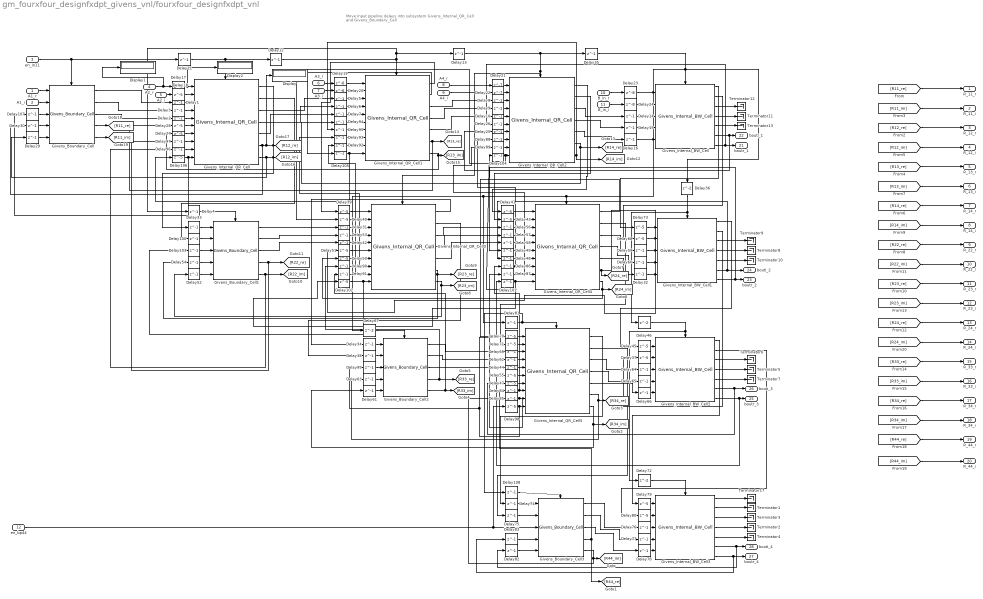
== system gm_fourxfour_designfxdpt_givens_vnl/fourxfour_designfxdpt_vnl ==
  note: Move Input pipeline delays into subsystem
      | Givens_Internal_QR_Cell and
      | Givens_Boundary_Cell
  "A1_r " : Inport
  A1_i : Inport  Port=2
  "en_in11 " : Inport  Port=3
  A2_r : Inport  Port=4
  A2_i : Inport  Port=5
  A3_r : Inport  Port=6
  A3_i : Inport  Port=7
  A4_r : Inport  Port=8
  A4_i : Inport  Port=9
  B_in_r : Inport  Port=10
  B_in_i : Inport  Port=11
  en_bp44 : Inport  Port=12
  Delay{1..16,25..26,29..35,38,42,44,48..49,52..54,56..66,69,74..78,81..97,99..101,103..105,107..108} (75 alike) : Delay  DelayLength=1  InitialCondition=0
  Delay{17..18,27..28,37,39..41,43,45,47,50..51,55,68,70..71,73,79..80,98,102,106} (23 alike) : Delay  DelayLength=5  InitialCondition=0
  Delay19 : Delay  DelayLength=6  InitialCondition=0
  Delay20 : Delay  DelayLength=6  InitialCondition=0
  Delay21 : Delay  DelayLength=7  InitialCondition=0
  Delay22 : Delay  DelayLength=7  InitialCondition=0
  Delay23 : Delay  DelayLength=8  InitialCondition=0
  Delay24 : Delay  DelayLength=8  InitialCondition=0
  Delay{36,46,67,72} (4 alike) : Delay  InitialCondition=0
  Display : Display
  Display1 : Display
  Display2 : Display
  Givens_Boundary_Cell{,1..3} (4 alike) : mylib/QR Components/Givens/Givens_Boundary_Cell  SystemSampleTime=-1
      settings: SourceProductName=QR_BW_block
  Givens_Internal_BW_Cell{,1..3} (4 alike) : mylib/QR Components/Givens/Givens_Internal_BW_Cell  SystemSampleTime=-1
      settings: SourceProductName=QR_BW_block
  Givens_Internal_QR_Cell{,1..5} (6 alike) : mylib/QR Components/Givens/Givens_Internal_QR_Cell  SystemSampleTime=-1
      settings: SourceProductName=QR_BW_block
  Terminator{1..13,17} (14 alike) : Terminator
  R_11_r : Outport
  R_11_i : Outport  Port=2
  R_12_r : Outport  Port=3
  R_12_i : Outport  Port=4
  R_13_r : Outport  Port=5
  R_13_i : Outport  Port=6
  R_14_r : Outport  Port=7
  R_14_i : Outport  Port=8
  R_22_r : Outport  Port=9
  R_22_i : Outport  Port=10
  R_23_r : Outport  Port=11
  R_23_i : Outport  Port=12
  R_24_r : Outport  Port=13
  R_24_i : Outport  Port=14
  R_33_r : Outport  Port=15
  R_33_i : Outport  Port=16
  R_34_r : Outport  Port=17
  R_34_i : Outport  Port=18
  R_44_r : Outport  Port=19
  R_44_i : Outport  Port=20
  boutr_1 : Outport  Port=21
  bouti_1 : Outport  Port=22
  boutr_2 : Outport  Port=23
  bouti_2 : Outport  Port=24
  boutr_3 : Outport  Port=25
  bouti_3 : Outport  Port=26
  boutr_4 : Outport  Port=27
  bouti_4 : Outport  Port=28
  wires:
  A2_r/1 -> Delay17/1, Display1/1
  Givens_Boundary_Cell/4 -> [R11_re]
  Givens_Boundary_Cell/5 -> [R11_im]
  [R11_re] -> R_11_r/1
  [R11_im] -> R_11_i/1
  [R12_re] -> R_12_r/1
  [R12_im] -> R_12_i/1
  [R13_re] -> R_13_r/1
  [R13_im] -> R_13_i/1
  [R14_re] -> R_14_r/1
  [R14_im] -> R_14_i/1
  [R22_re] -> R_22_r/1
  [R22_im] -> R_22_i/1
  [R23_im] -> R_23_i/1
  [R23_re] -> R_23_r/1
  [R24_re] -> R_24_r/1
  [R24_im] -> R_24_i/1
  [R33_im] -> R_33_i/1
  [R33_re] -> R_33_r/1
  [R34_im] -> R_34_i/1
  [R34_re] -> R_34_r/1
  [R44_re] -> R_44_r/1
  [R44_im] -> R_44_i/1
  Delay108/1 -> Givens_Boundary_Cell3/Enable
  Delay107/1 -> Givens_Boundary_Cell/3
  Delay103/1 -> Givens_Boundary_Cell1/3
  Delay99/1 -> Givens_Boundary_Cell2/3
  Delay72/1 -> Givens_Internal_BW_Cell3/Enable
  Delay46/1 -> Givens_Internal_BW_Cell2/Enable, Delay72/1
  Delay81/1 -> Delay108/1, Givens_Internal_QR_Cell5/Enable
  Delay36/1 -> Givens_Internal_BW_Cell1/Enable, Delay46/1
  Delay35/1 -> Givens_Internal_QR_Cell4/Enable, Delay67/1, Delay81/1, Delay36/1, Givens_Internal_BW_Cell/Enable
  Delay11/1 -> Delay12/1, Givens_Internal_QR_Cell/Enable
  Delay13/1 -> Givens_Internal_QR_Cell2/Enable, Givens_Internal_QR_Cell3/Enable, Delay35/1
  Delay12/1 -> Givens_Internal_QR_Cell1/Enable, Delay13/1, Delay4/1
  Delay4/1 -> Givens_Boundary_Cell1/Enable
  "en_in11 "/1 -> Delay11/1, Givens_Boundary_Cell/Enable
  Givens_Internal_QR_Cell1/1 -> Delay39/1
  Givens_Internal_QR_Cell1/2 -> Delay40/1
  Givens_Internal_BW_Cell1/6 -> Delay48/1, bouti_2/1
  Givens_Internal_BW_Cell1/7 -> Delay49/1, boutr_2/1
  Givens_Internal_BW_Cell/5 -> Terminator13/1
  Givens_Internal_BW_Cell/3 -> Terminator12/1
  Givens_Internal_BW_Cell/4 -> Terminator11/1
  Givens_Internal_BW_Cell1/5 -> Terminator10/1
  Givens_Internal_BW_Cell1/3 -> Terminator9/1
  Givens_Internal_BW_Cell1/4 -> Terminator8/1
  Givens_Internal_BW_Cell2/5 -> Terminator7/1
  Givens_Internal_BW_Cell2/4 -> Terminator5/1
  Givens_Internal_BW_Cell2/3 -> Terminator6/1
  Delay100/1 -> Givens_Boundary_Cell1/2
  Givens_Internal_QR_Cell/2 -> Delay100/1
  Delay48/1 -> Givens_Internal_QR_Cell4/7
  Delay105/1 -> Givens_Internal_QR_Cell1/10, Delay106/1
  Delay101/1 -> Givens_Internal_QR_Cell4/10, Delay102/1, Delay104/1
  Delay104/1 -> Givens_Internal_QR_Cell2/10, Delay105/1
  Delay98/1 -> Givens_Internal_QR_Cell5/10, Delay99/1, Delay101/1
  Delay97/1 -> Givens_Internal_QR_Cell/8
  Delay96/1 -> Givens_Internal_QR_Cell/9
  Delay95/1 -> Givens_Internal_QR_Cell1/7
  Delay94/1 -> Givens_Internal_QR_Cell1/6
  Delay93/1 -> Givens_Internal_QR_Cell1/8
  Delay92/1 -> Givens_Internal_QR_Cell1/9
  Delay91/1 -> Delay92/1, Givens_Internal_QR_Cell3/9
  Delay90/1 -> Givens_Internal_QR_Cell3/8, Delay93/1
  Delay89/1 -> Givens_Internal_QR_Cell2/9
  Delay88/1 -> Givens_Internal_QR_Cell2/8
  Delay87/1 -> Delay89/1, Givens_Internal_QR_Cell4/9
  Delay86/1 -> Givens_Internal_QR_Cell4/8, Delay88/1
  Delay85/1 -> Givens_Internal_QR_Cell5/9, Delay87/1
  Delay84/1 -> Givens_Internal_QR_Cell5/8, Delay86/1
  Givens_Internal_BW_Cell3/5 -> Terminator4/1
  Givens_Internal_BW_Cell3/3 -> Terminator3/1
  Givens_Internal_BW_Cell3/4 -> Terminator2/1
  Givens_Internal_BW_Cell3/2 -> Terminator1/1
  Givens_Internal_BW_Cell3/1 -> Terminator17/1
  Givens_Boundary_Cell3/4 -> [R44_re], Delay84/1
  Givens_Boundary_Cell3/5 -> Delay85/1, [R44_im]
  Delay83/1 -> Givens_Boundary_Cell3/4
  Delay82/1 -> Givens_Boundary_Cell3/5
  Givens_Internal_BW_Cell3/6 -> Delay82/1, bouti_4/1
  Givens_Internal_BW_Cell3/7 -> boutr_4/1, Delay83/1
  Delay80/1 -> Givens_Internal_BW_Cell3/2
  Givens_Internal_BW_Cell2/2 -> Delay80/1
  Delay79/1 -> Givens_Internal_BW_Cell3/1
  Givens_Internal_BW_Cell2/1 -> Delay79/1
  Delay78/1 -> Givens_Internal_BW_Cell3/5
  Delay77/1 -> Givens_Internal_BW_Cell3/4
  Delay76/1 -> Givens_Internal_BW_Cell3/3
  Givens_Boundary_Cell3/3 -> Delay78/1
  Givens_Boundary_Cell3/2 -> Delay77/1
  Givens_Boundary_Cell3/1 -> Delay76/1
  en_bp44/1 -> Delay98/1, Givens_Boundary_Cell3/3
  Delay75/1 -> Givens_Boundary_Cell3/2
  Delay74/1 -> Givens_Boundary_Cell3/1
  Givens_Internal_QR_Cell5/2 -> Delay75/1
  Givens_Internal_QR_Cell5/1 -> Delay74/1
  Delay73/1 -> Givens_Internal_BW_Cell1/1
  Delay68/1 -> Givens_Internal_BW_Cell1/2
  Givens_Internal_BW_Cell/2 -> Delay68/1
  Givens_Internal_BW_Cell/1 -> Delay73/1
  Delay67/1 -> Givens_Boundary_Cell2/Enable
  Givens_Internal_BW_Cell2/6 -> bouti_3/1, Delay47/1
  Givens_Internal_BW_Cell2/7 -> boutr_3/1, Delay55/1
  Delay45/1 -> Givens_Internal_BW_Cell2/1
  Delay37/1 -> Givens_Internal_BW_Cell2/2
  Givens_Internal_BW_Cell1/2 -> Delay37/1
  Givens_Internal_BW_Cell1/1 -> Delay45/1
  Delay71/1 -> Givens_Internal_QR_Cell5/2
  Delay70/1 -> Givens_Internal_QR_Cell5/1
  Givens_Internal_QR_Cell4/2 -> Delay71/1
  Givens_Internal_QR_Cell4/1 -> Delay70/1
  Delay69/1 -> Givens_Internal_QR_Cell5/3
  Givens_Boundary_Cell2/2 -> Delay62/1
  Givens_Boundary_Cell2/1 -> Delay69/1
  Delay38/1 -> Givens_Boundary_Cell2/2
  Delay34/1 -> Givens_Boundary_Cell2/1
  Givens_Internal_QR_Cell3/2 -> Delay38/1
  Givens_Internal_QR_Cell3/1 -> Delay34/1
  Givens_Boundary_Cell2/4 -> Delay90/1, [R33_re]
  Givens_Internal_QR_Cell5/6 -> Delay63/1, [R34_re]
  Delay64/1 -> Givens_Internal_BW_Cell2/3
  Delay47/1 -> Givens_Internal_QR_Cell5/7
  Delay61/1 -> Givens_Boundary_Cell2/5
  Delay62/1 -> Givens_Internal_QR_Cell5/4
  Givens_Internal_QR_Cell5/5 -> Delay66/1
  Givens_Boundary_Cell2/5 -> [R33_im], Delay91/1
  Delay44/1 -> Givens_Internal_QR_Cell5/5
  Givens_Internal_QR_Cell5/4 -> Delay65/1
  Delay65/1 -> Givens_Internal_BW_Cell2/4
  Givens_Boundary_Cell2/3 -> Delay44/1
  Givens_Internal_QR_Cell5/3 -> Delay64/1
  Delay55/1 -> Givens_Internal_QR_Cell5/6
  Delay66/1 -> Givens_Internal_BW_Cell2/5
  Givens_Internal_QR_Cell5/7 -> [R34_im], Delay61/1
  Delay63/1 -> Givens_Boundary_Cell2/4
  Delay49/1 -> Givens_Internal_QR_Cell4/6
  Givens_Internal_QR_Cell2/7 -> [R14_im], Delay95/1
  Givens_Internal_QR_Cell2/6 -> [R14_re], Delay94/1
  Delay25/1 -> Givens_Internal_QR_Cell2/7
  Delay26/1 -> Givens_Internal_QR_Cell2/6
  Delay102/1 -> Delay103/1, Givens_Internal_QR_Cell3/10
  Delay33/1 -> Givens_Boundary_Cell1/1
  Delay32/1 -> Givens_Internal_BW_Cell1/5
  Delay40/1 -> Givens_Internal_QR_Cell3/2
  Givens_Internal_QR_Cell2/1 -> Delay41/1
  Delay58/1 -> Givens_Internal_QR_Cell4/5
  Delay51/1 -> Givens_Internal_QR_Cell3/6
  Delay59/1 -> Givens_Internal_BW_Cell1/3
  Delay43/1 -> Givens_Internal_QR_Cell4/2
  Delay41/1 -> Givens_Internal_QR_Cell4/1
  Givens_Boundary_Cell1/1 -> Delay31/1
  Givens_Internal_QR_Cell3/3 -> Delay56/1
  Delay60/1 -> Givens_Internal_BW_Cell1/4
  Givens_Boundary_Cell1/4 -> Delay97/1, [R22_re]
  Givens_Boundary_Cell1/3 -> Delay42/1
  Givens_Boundary_Cell1/2 -> Delay53/1
  Delay31/1 -> Givens_Internal_QR_Cell3/3
  Givens_Internal_QR_Cell3/6 -> Delay54/1, [R23_re]
  Delay57/1 -> Givens_Internal_QR_Cell4/4
  Delay52/1 -> Givens_Boundary_Cell1/5
  Givens_Internal_QR_Cell3/4 -> Delay57/1
  Givens_Internal_QR_Cell3/5 -> Delay58/1
  Givens_Internal_QR_Cell2/2 -> Delay43/1
  Delay53/1 -> Givens_Internal_QR_Cell3/4
  Delay56/1 -> Givens_Internal_QR_Cell4/3
  Givens_Boundary_Cell1/5 -> Delay96/1, [R22_im]
  Delay42/1 -> Givens_Internal_QR_Cell3/5
  Delay39/1 -> Givens_Internal_QR_Cell3/1
  Givens_Internal_QR_Cell/1 -> Delay33/1
  Delay50/1 -> Givens_Internal_QR_Cell3/7
  Givens_Internal_QR_Cell4/5 -> Delay32/1
  Givens_Internal_QR_Cell4/6 -> [R24_re], Delay51/1
  Givens_Internal_QR_Cell4/7 -> [R24_im], Delay50/1
  Givens_Internal_QR_Cell4/4 -> Delay60/1
  Givens_Internal_QR_Cell4/3 -> Delay59/1
  Delay54/1 -> Givens_Boundary_Cell1/4
  Givens_Internal_QR_Cell3/7 -> [R23_im], Delay52/1
  Delay30/1 -> Givens_Boundary_Cell/4
  Delay29/1 -> Givens_Boundary_Cell/5
  Delay28/1 -> Givens_Internal_QR_Cell/6
  Delay27/1 -> Givens_Internal_QR_Cell/7
  Givens_Internal_BW_Cell/7 -> boutr_1/1, Delay26/1
  Givens_Internal_BW_Cell/6 -> bouti_1/1, Delay25/1
  Delay24/1 -> Givens_Internal_BW_Cell/2
  Delay23/1 -> Givens_Internal_BW_Cell/1
  Delay22/1 -> Givens_Internal_QR_Cell2/2
  Delay21/1 -> Givens_Internal_QR_Cell2/1
  Delay20/1 -> Givens_Internal_QR_Cell1/2
  Delay19/1 -> Givens_Internal_QR_Cell1/1
  Delay18/1 -> Givens_Internal_QR_Cell/2
  Delay17/1 -> Givens_Internal_QR_Cell/1, Display2/1
  Delay16/1 -> Givens_Internal_BW_Cell/5
  Delay15/1 -> Givens_Internal_BW_Cell/4
  Delay14/1 -> Givens_Internal_BW_Cell/3
  Givens_Internal_QR_Cell2/5 -> Delay16/1
  Givens_Internal_QR_Cell2/4 -> Delay15/1
  Givens_Internal_QR_Cell2/3 -> Delay14/1
  B_in_i/1 -> Delay24/1
  B_in_r/1 -> Delay23/1
  Delay10/1 -> Givens_Internal_QR_Cell2/5
  A4_r/1 -> Delay21/1
  Givens_Internal_QR_Cell1/5 -> Delay10/1
  Givens_Internal_QR_Cell1/6 -> Delay28/1, [R13_re]
  Delay9/1 -> Givens_Internal_QR_Cell2/4
  Givens_Internal_QR_Cell1/3 -> Delay8/1
  Delay8/1 -> Givens_Internal_QR_Cell2/3
  Givens_Internal_QR_Cell1/4 -> Delay9/1
  A4_i/1 -> Delay22/1
  Givens_Internal_QR_Cell1/7 -> [R13_im], Delay27/1
  A3_r/1 -> Delay19/1
  A3_i/1 -> Delay20/1
  Givens_Internal_QR_Cell/7 -> [R12_im], Delay29/1
  Givens_Internal_QR_Cell/6 -> Delay30/1, [R12_re], Display/1
  Delay7/1 -> Givens_Internal_QR_Cell1/5
  Delay6/1 -> Givens_Internal_QR_Cell1/4
  Delay5/1 -> Givens_Internal_QR_Cell1/3
  Givens_Internal_QR_Cell/5 -> Delay7/1
  Givens_Internal_QR_Cell/4 -> Delay6/1
  Givens_Internal_QR_Cell/3 -> Delay5/1
  A2_i/1 -> Delay18/1
  Delay106/1 -> Givens_Internal_QR_Cell/10, Delay107/1
  A1_i/1 -> Givens_Boundary_Cell/2
  "A1_r "/1 -> Givens_Boundary_Cell/1
  Delay2/1 -> Givens_Internal_QR_Cell/5
  Delay1/1 -> Givens_Internal_QR_Cell/3
  Delay3/1 -> Givens_Internal_QR_Cell/4
  Givens_Boundary_Cell/3 -> Delay2/1
  Givens_Boundary_Cell/2 -> Delay3/1
  Givens_Boundary_Cell/1 -> Delay1/1
